simulink model "getnsave_data_infra_trans"  (Simulink 7.4)
settings: Solver=FixedStepDiscrete  StartTime=0.0  StopTime=inf  FixedStep=0.004  RelTol=1e-3
values from neighbouring files (symbols this model uses):
  B = Rand_trials    [init_Traj_expe_2.m]
  n = length(MT_0370027B_0010x2D000)-5    [ReadDataFromIMU.m]    (also in infralim_random_values2.m = length(Trial_matrix); init_Traj_expe_2.m = 1)
libraries: instrumentlib x1, xpclib x1
settings Model: Creator=iMose1  LastModifiedBy=iMose1

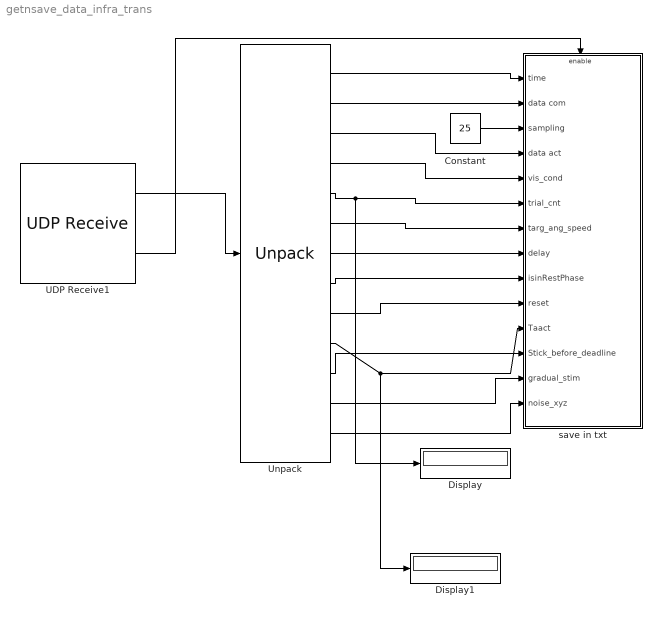
== system getnsave_data_infra_trans ==
  Constant : Constant  Value=25  OutDataType=fixdt(1, 16)  OutScaling=2^0
  Display : Display
  Display1 : Display
  UDP Receive1 : instrumentlib/UDP Receive  DialogController=instrumentcreatedialog  DialogControllerArgs=DataTag0  Host=192.168.102.111  Port=9250  LocalPort=9250  DataSize=100  EnableBlockingMode=off  Timeout=10  SampleTime=0.004  DataType=uint8  ByteOrder=BigEndian
  Unpack : xpclib/UDP/Unpack  dimensions={1,3,3,1,1,3,1,1,1,1,3,3,3}  datatypes={'single','single','single','single','single','single','single','single','single','single','single','single','single'}  byteAlign=1
  save in txt : Subsystem
  wires:
  UDP Receive1/1 -> Unpack/1
  Unpack/1 -> save in txt/1(time)
  Unpack/2 -> save in txt/2(data com)
  Constant/1 -> save in txt/3(sampling)
  UDP Receive1/2 -> save in txt/Enable
  Unpack/9 -> save in txt/10(reset)
  Unpack/8 -> save in txt/9(isinRestPhase)
  Unpack/7 -> save in txt/8(delay)
  Unpack/6 -> save in txt/7(targ_ang_speed)
  Unpack/5 -> save in txt/6(trial_cnt), Display/1
  Unpack/3 -> save in txt/4(data act)
  Unpack/4 -> save in txt/5(vis_cond)
  Unpack/10 -> save in txt/11(Taact), Display1/1
  Unpack/11 -> save in txt/12(Stick_before_deadline)
  Unpack/12 -> save in txt/13(gradual_stim)
  Unpack/13 -> save in txt/14(noise_xyz)

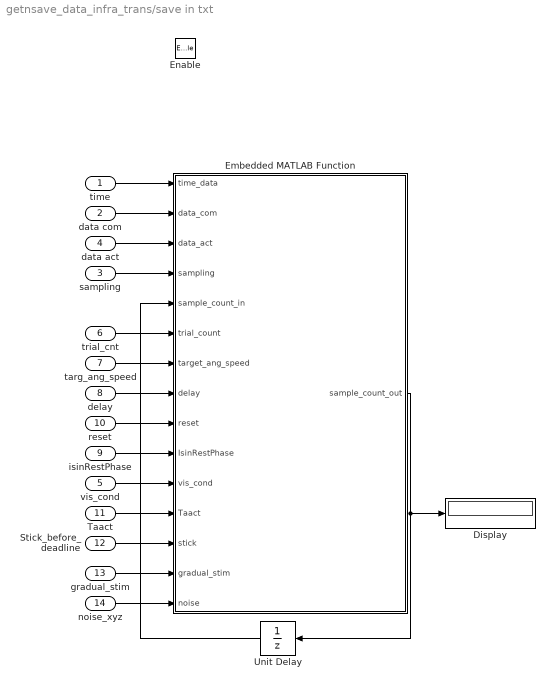
== system getnsave_data_infra_trans/save in txt ==
  time : Inport
  data com : Inport  Port=2
  sampling : Inport  Port=3
  data act : Inport  Port=4
  vis_cond : Inport  Port=5
  trial_cnt : Inport  Port=6
  targ_ang_speed : Inport  Port=7
  delay : Inport  Port=8
  isinRestPhase : Inport  Port=9
  reset : Inport  Port=10
  Taact : Inport  Port=11
  Stick_before_deadline : Inport  Port=12
  gradual_stim : Inport  Port=13
  noise_xyz : Inport  Port=14
  Enable : EnablePort  ShowOutputPort=on
  Display : Display
  Embedded MATLAB Function : Stateflow chart
  Unit Delay : UnitDelay  X0=1  SampleTime=-1
  wires:
  Embedded MATLAB Function/1(sample_count_out) -> Unit Delay/1, Display/1
  Unit Delay/1 -> Embedded MATLAB Function/5(sample_count_in)
  time/1 -> Embedded MATLAB Function/1(time_data)
  data com/1 -> Embedded MATLAB Function/2(data_com)
  sampling/1 -> Embedded MATLAB Function/4(sampling)
  trial_cnt/1 -> Embedded MATLAB Function/6(trial_count)
  targ_ang_speed/1 -> Embedded MATLAB Function/7(target_ang_speed)
  delay/1 -> Embedded MATLAB Function/8(delay)
  reset/1 -> Embedded MATLAB Function/9(reset)
  isinRestPhase/1 -> Embedded MATLAB Function/10(IsinRestPhase)
  vis_cond/1 -> Embedded MATLAB Function/11(vis_cond)
  data act/1 -> Embedded MATLAB Function/3(data_act)
  Taact/1 -> Embedded MATLAB Function/12(Taact)
  Stick_before_deadline/1 -> Embedded MATLAB Function/13(stick)
  gradual_stim/1 -> Embedded MATLAB Function/14(gradual_stim)
  noise_xyz/1 -> Embedded MATLAB Function/15(noise)

== matlab function save in txt/Embedded MATLAB Function ==
  data: time_data input double; sample_count_out output double; data_com input double; data_act input double; sampling input double; sample_count_in input double; trial_count input double; target_ang_speed input double; delay input double; reset input double; IsinRestPhase input double; vis_cond input double; B parameter double; n parameter double; Taact input double; stick input double; gradual_stim input double; noise input double
function sample_count_out  = save_data(time_data,data_com,data_act,sampling,sample_count_in,trial_count,target_ang_speed,delay,reset,IsinRestPhase,vis_cond,B,n,Taact,stick,gradual_stim,noise)
%#eml
eml.extrinsic('fopen')
eml.extrinsic('fclose')
eml.extrinsic('fprintf')
eml.extrinsic('sprintf')

if(reset)
    sample_count_in=1;
end



if(IsinRestPhase)
    sample_count_out=sample_count_in;
else
    if sample_count_in==sampling
        index=B(trial_count,4);
        
        %fileID=fopen('subject1.txt','a+');
        fileID=fopen(sprintf('subject%i.txt',n),'a+');
        fprintf(fileID,'%f\t%f\t%f\t%f\t%f\t%f\t%f\t%f\t%f\t%f\t%f\t%f\t%f\t%f\t%f\t%f\t%f\t%f\t%f\t%f\t%f\t%f\r\n', trial_count, time_data, data_com(1), data_com(2), data_com(3), data_act(1),data_act(2),data_act(3), delay, target_ang_speed(1), target_ang_speed(2), target_ang_speed(3), vis_cond, index, Taact,stick(1),stick(2),stick(3),gradual_stim(index),noise(1),noise(2),noise(3)); %save 3 axes from data_com and data_act
        %fprintf(fileID,'%f\t%f\t%f\t%f\t%f\t%f\t%f\t%f\t%f\t%f\r\n', trial_count, time_data, data_com(1), data_com(2), data_com(3), delay, target_ang_speed(1), target_ang_speed(2), target_ang_speed(3), vis_cond);%save three axes from data
        fclose(fileID);
        
        sample_count_out=1;
    else
        sample_count_out=sample_count_in+1;
    end
end

end
